simulink model "Int_Cost"  (R2016b)
settings: Solver=VariableStepAuto  StartTime=0.0  StopTime=1000  RelTol=1e-3
values from neighbouring files (symbols this model uses):
  a1 = 50    [a_init.m]
  a2 = -1    [a_init.m]
  b = 1    [a_init.m]
  beta = 0.1    [a_init.m]
  G = [5000 500 500]    [a_init.m]
  ms = [1 p 2*p]    [a_init.m]
  t0 = [18 4 1]    [a_init.m]
  Ue = 0.4977    [a_init.m]
  Ye = 0.7313    [a_init.m]
libraries: simulink x1
settings Model: Creator=Niels  LastModifiedBy=Niels

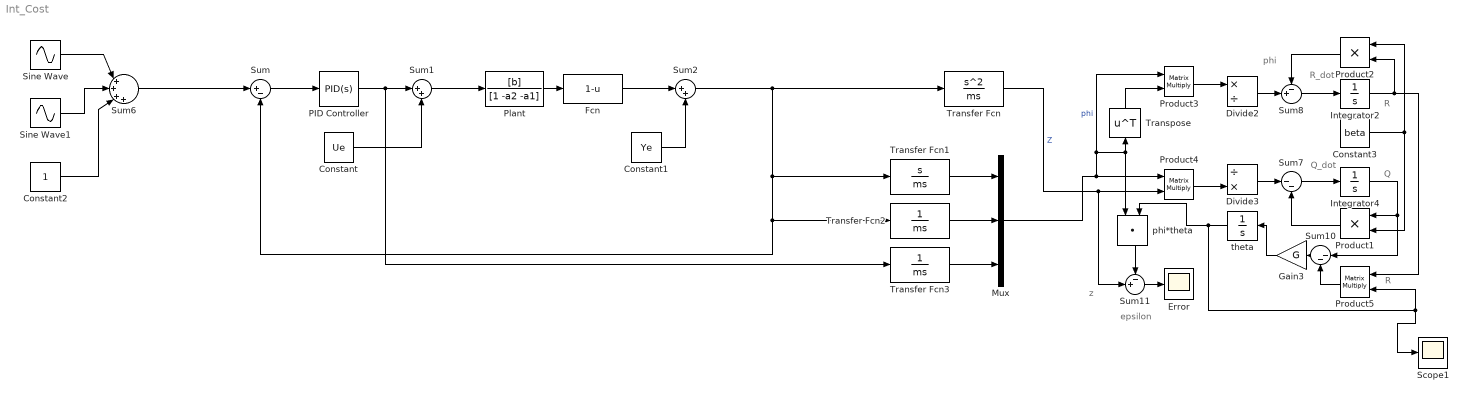
== system Int_Cost ==
  note: R
  note: z
  note: R
  note: Q
  note: R_dot
  note: Q_dot
  note: epsilon
  note: phi
  Constant : Constant  Value=Ue
  Constant1 : Constant  Value=Ye
  Constant2 : Constant
  Constant3 : Constant  Value=beta
  Divide2 : Product  Inputs=*/
  Divide3 : Product  Inputs=/*
  Error : Scope
  Fcn : Fcn  Expr=1-u
  Gain3 : Gain  Gain=G
  Integrator2 : Integrator
  Integrator4 : Integrator
  Mux : Mux  Inputs=3
  PID Controller : simulink/Continuous/PID Controller  Controller=PID  TimeDomain=Continuous-time  SampleTime=-1  IntegratorMethod=Forward Euler  FilterMethod=Forward Euler  Form=Parallel  UseFilter=on  ControllerParametersSource=internal  P=0.7  I=0.15  D=0.04  N=100  InitialConditionSource=internal  InitialConditionForIntegrator=0  InitialConditionForFilter=0  ExternalReset=none  LimitOutput=off  UpperSaturationLimit=inf  LowerSaturationLimit=-inf  LinearizeAsGain=on  AntiWindupMode=none  Kb=1  TrackingMode=off  Kt=1  PParamMin=[]  PParamMax=[]  IParamMin=[]  IParamMax=[]  DParamMin=[]  DParamMax=[]  NParamMin=[]  NParamMax=[]  KbParamMin=[]  KbParamMax=[]  KtParamMin=[]  KtParamMax=[]  POutMin=[]  POutMax=[]  IOutMin=[]  IOutMax=[]  DOutMin=[]  DOutMax=[]  NOutMin=[]  NOutMax=[]  KbOutMin=[]  KbOutMax=[]  KtOutMin=[]  KtOutMax=[]  IntegratorOutMin=[]  IntegratorOutMax=[]  FilterOutMin=[]  FilterOutMax=[]  SumOutMin=[]  SumOutMax=[]  SumI1OutMin=[]  SumI1OutMax=[]  SumI2OutMin=[]  SumI2OutMax=[]  SumI3OutMin=[]  SumI3OutMax=[]  SumDOutMin=[]  SumDOutMax=[]  SaturationOutMin=[]  SaturationOutMax=[]  IntegratorContinuousStateAttributes=''  IntegratorStateMustResolveToSignalObject=off  IntegratorRTWStateStorageClass=Auto  FilterContinuousStateAttributes=''  FilterStateMustResolveToSignalObject=off  FilterRTWStateStorageClass=Auto  DifferentiatorICPrevScaledInput=0  DifferentiatorOutMin=[]  DifferentiatorOutMax=[]
  Plant : TransferFcn  Numerator=[b]  Denominator=[1 -a2 -a1]
  Product1 : Product
  Product2 : Product
  Product3 : Product  Inputs=**  Multiplication=Matrix(*)
  Product4 : Product  Inputs=**  Multiplication=Matrix(*)
  Product5 : Product  Multiplication=Matrix(*)
  Scope1 : Scope
  Sine Wave : Sin  SampleTime=0
  Sine Wave1 : Sin  SampleTime=0
  Sum : Sum  Inputs=|+-
  Sum1 : Sum  Inputs=|++
  Sum10 : Sum  Inputs=|--
  Sum11 : Sum  Inputs=-+|
  Sum2 : Sum  Inputs=|++
  Sum6 : Sum  Inputs=|++++
  Sum7 : Sum  Inputs=|--
  Sum8 : Sum  Inputs=-+|
  Transfer Fcn : TransferFcn  Numerator=[1 0 0]  Denominator=ms
  Transfer Fcn1 : TransferFcn  Numerator=[1 0]  Denominator=ms
  Transfer Fcn2 : TransferFcn  Denominator=ms
  Transfer Fcn3 : TransferFcn  Denominator=ms
  Transpose : Math  Operator=transpose  SaturateOnIntegerOverflow=on
  phi*theta : DotProduct  InputSameDT=on  OutDataTypeStr=Inherit: Inherit via internal rule
  theta : Integrator  InitialCondition=t0
  wires:
  Sum6/1 -> Sum/1
  Sum/1 -> PID Controller/1
  PID Controller/1 -> Transfer Fcn3/1, Sum1/1
  Constant/1 -> Sum1/2
  Sum1/1 -> Plant/1
  Plant/1 -> Fcn/1
  Constant1/1 -> Sum2/2
  Fcn/1 -> Sum2/1
  Sum2/1 -> Transfer Fcn/1, Transfer Fcn1/1, Transfer Fcn2/1, Sum/2
  Transfer Fcn1/1 -> Mux/1
  Transfer Fcn2/1 -> Mux/2
  Transfer Fcn3/1 -> Mux/3
  Transfer Fcn/1 -> Sum11/2, Product4/2  "Z"
  Mux/1 -> phi*theta/1, Transpose/1, Product3/1, Product4/1  "phi"
  Sine Wave/1 -> Sum6/1
  Sine Wave1/1 -> Sum6/2
  Constant2/1 -> Sum6/3
  Integrator2/1 -> Product5/1, Product2/2
  phi*theta/1 -> Sum11/1
  Constant3/1 -> Product1/2, Product2/1
  Gain3/1 -> theta/1
  theta/1 -> Scope1/1, Product5/2, phi*theta/2
  Transpose/1 -> Product3/2
  Integrator4/1 -> Sum10/1, Product1/1
  Sum7/1 -> Integrator4/1
  Sum11/1 -> Error/1
  Divide2/1 -> Sum8/2
  Product3/1 -> Divide2/1
  Sum10/1 -> Gain3/1
  Product4/1 -> Divide3/2
  Product5/1 -> Sum10/2
  Product1/1 -> Sum7/2
  Product2/1 -> Sum8/1
  ? -> Divide2/2, Divide3/1
  Divide3/1 -> Sum7/1
  Sum8/1 -> Integrator2/1
